simulink model "Lab5_PostLablul"  (R2021b)
settings: Solver=VariableStepAuto  StartTime=0.0  StopTime=10.0  RelTol=1e-3
libraries: spsDCMachineLib x2, spsDCVoltageSourceLib x2, spspowerguiLib x1
settings Model: Creator=Dell  LastModifiedBy=Dell

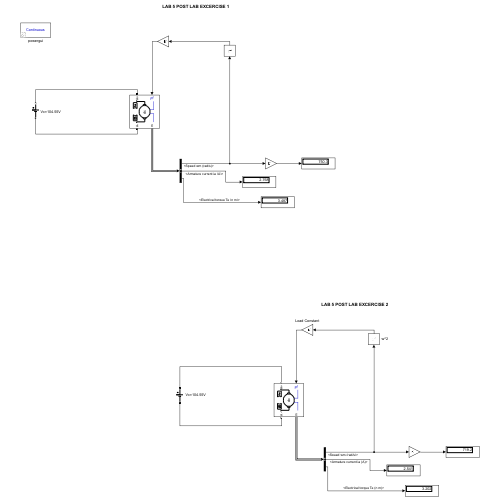
[thumbnail: Simulink's stored preview of the top-level diagram]
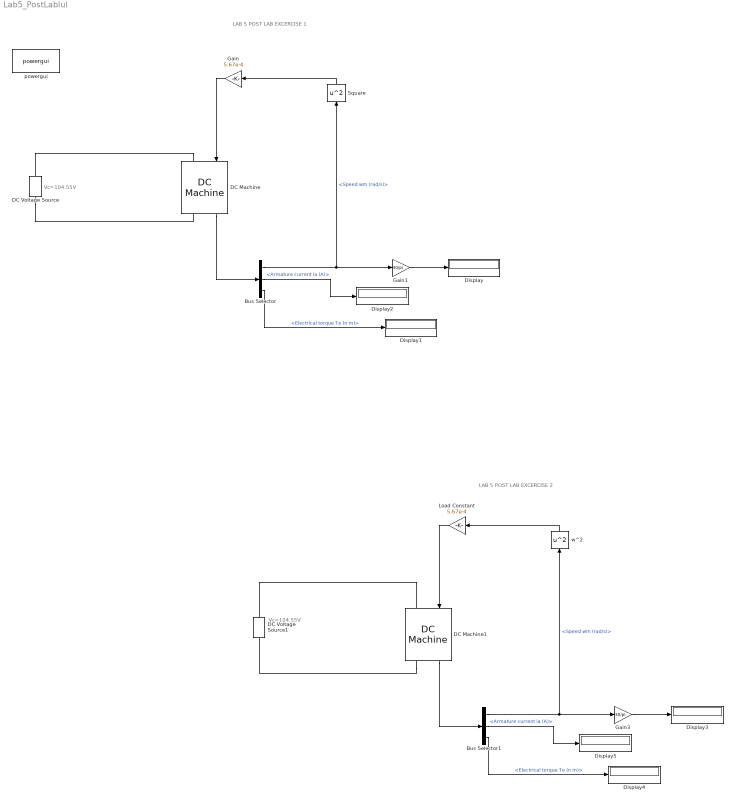
== system Lab5_PostLablul ==
  note: LAB 5 POST LAB EXCERCISE 1
  note: Vc=104.55V
  note: LAB 5 POST LAB EXCERCISE 2
  note: Vc=104.55V
  Bus Selector : BusSelector  OutputSignals=Speed wm (rad/s),Armature current ia (A),Electrical torque Te (n m)
  Bus Selector1 : BusSelector  OutputSignals=Speed wm (rad/s),Armature current ia (A),Electrical torque Te (n m)
  DC Machine : spsDCMachineLib/DC Machine  PresetModel=No  MechanicalLoad=Torque TL  FieldType=Permanent magnet  ShowDetailedParameters=on  MeasurementBus=off  RLa="[ 2.0  0.011]"  RLf="[ 240  120]"  Laf=1.8  MachineConstant=Torque constant (N.m/A)  Ke=1.8  Kt=1.26  J=0.05  Bm=0  Tf=0  w0=1  Ifinit=1  TsPowergui=0  TsBlock=-1
  DC Machine1 : spsDCMachineLib/DC Machine  PresetModel=No  MechanicalLoad=Torque TL  FieldType=Permanent magnet  ShowDetailedParameters=on  MeasurementBus=off  RLa="[ 2.0  0.011]"  RLf="[ 240  120]"  Laf=1.8  MachineConstant=Torque constant (N.m/A)  Ke=1.8  Kt=1.26  J=0.05  Bm=0  Tf=0  w0=1  Ifinit=1  TsPowergui=0  TsBlock=-1
  DC Voltage Source : spsDCVoltageSourceLib/DC Voltage Source  Amplitude=104.55  Measurements=Voltage
  DC Voltage Source1 : spsDCVoltageSourceLib/DC Voltage Source  Amplitude=100  Measurements=None
  Display{,1..5} (6 alike) : Display
  Gain : Gain  Gain=5.67e-4
  Gain1 : Gain  Gain=30/pi
  Gain3 : Gain  Gain=30/pi
  Load Constant : Gain  Gain=5.67e-4
  Square : Math  Operator=square  SaturateOnIntegerOverflow=on
  powergui : spspowerguiLib/powergui  Priority=1  SimulationMode=Continuous  SampleTime=50e-6  frequency=60  Iterations=50  frequencyindice=0  Pbase=100e6  ErrMax=1e-4  UnitsV=kV  UnitsW=MW  buscounter=0  FunctionMessages=off  echomessages=off  EnableUseOfTLC=off  CurrentSourceSwitches=off  DisableSnubberDevices=off  DisableRonSwitches=off  DisableVfSwitches=off  DisplayEquations=off  AutomaticDiscreteSolvers=off  SolverType=Tustin/Backward Euler (TBE)  Interpol=off  ExternalGateDelay=off  methode=off  Ts=100  x0status=blocks  SPID=on  SwTol=0  HookPort=off  NonlinearTolerance=1e-4  nMaxIteration=100  ContinueOnMaxIteration=off  RestoreLinks=warning  ResistiveCurrentMeasurement=off  Frange=[0:2:500]  Ylog=off  Xlog=on  ShowGrid=off  save=off  variable=ZData  structure=0  ZoomFFT=off  StartTime=0.0  cycles=1  DisplayStyle=1  fundamental=60  FreqAxis=off  MaxFrequency=1000  frequencyindicesteady=1  RmsSteady=1  display=off
  w^2 : Math  Operator=square  SaturateOnIntegerOverflow=on
  wires:
  DC Machine/1 -> Bus Selector/1
  Bus Selector/1 -> Gain1/1, Square/1  "<Speed wm (rad/s)>"
  Bus Selector/2 -> Display2/1  "<Armature current ia (A)>"
  Bus Selector/3 -> Display1/1  "<Electrical torque Te (n m)>"
  Square/1 -> Gain/1
  Gain/1 -> DC Machine/1
  Gain1/1 -> Display/1
  Gain3/1 -> Display3/1
  Bus Selector1/2 -> Display5/1  "<Armature current ia (A)>"
  Bus Selector1/3 -> Display4/1  "<Electrical torque Te (n m)>"
  Bus Selector1/1 -> Gain3/1, w^2/1  "<Speed wm (rad/s)>"
  w^2/1 -> Load Constant/1
  Load Constant/1 -> DC Machine1/1
  DC Machine1/1 -> Bus Selector1/1
  connections:
  DC Voltage Source/RConn1 -- DC Machine/LConn1
  DC Voltage Source/LConn1 -- DC Machine/RConn1
  DC Machine1/RConn1 -- DC Voltage Source1/LConn1
  DC Voltage Source1/RConn1 -- DC Machine1/LConn1
